simulink model "model_cl"  (R2019b)
settings: Solver=VariableStepAuto  StartTime=0.0  StopTime=100  RelTol=1e-3
settings Model: Creator=rcc  LastModifiedBy=rcc

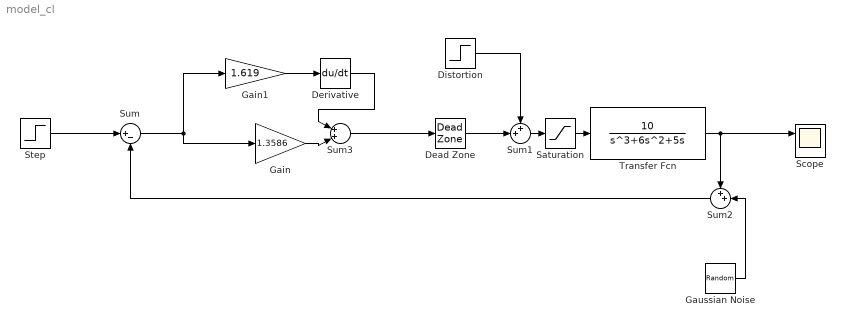
== system model_cl ==
  Dead Zone : DeadZone  LowerValue=-1  UpperValue=1  SaturateOnIntegerOverflow=on
  Derivative : Derivative
  Distortion : Step  Time=15  After=0.1  SampleTime=0
  Gain : Gain  Gain=1.3586
  Gain1 : Gain  Gain=1.619
  Gaussian Noise : RandomNumber  Seed=1  SampleTime=0.1
  Saturation : Saturate
  Scope : Scope  NumInputPorts=2
  Step : Step  SampleTime=0
  Sum : Sum  Inputs=|+-
  Sum1 : Sum  Inputs=++|
  Sum2 : Sum  Inputs=++|
  Sum3 : Sum  Inputs=|++|
  Transfer Fcn : TransferFcn  Numerator=[10]  Denominator=[1 6 5 0]
  wires:
  Transfer Fcn/1 -> Sum2/1, Scope/1
  Step/1 -> Sum/1
  Distortion/1 -> Sum1/1
  Sum2/1 -> Sum/2
  Dead Zone/1 -> Sum1/2
  Gain/1 -> Sum3/2
  Derivative/1 -> Sum3/1
  Gain1/1 -> Derivative/1
  Sum3/1 -> Dead Zone/1
  Sum/1 -> Gain/1, Gain1/1
  Gaussian Noise/1 -> Sum2/2
  Sum1/1 -> Saturation/1
  Saturation/1 -> Transfer Fcn/1
